simulink model "crne"  (R2018b)
settings: Solver=VariableStepAuto  StartTime=0.0  StopTime=7  RelTol=1e-3
undefined symbols (not defined in the file): eff_g_y, eff_m_y, J_phi, Kg_y, Kt_y, mp, r_y_reel
libraries: fuzblock x1
settings Model: Creator=EMiR  LastModifiedBy=EMiR

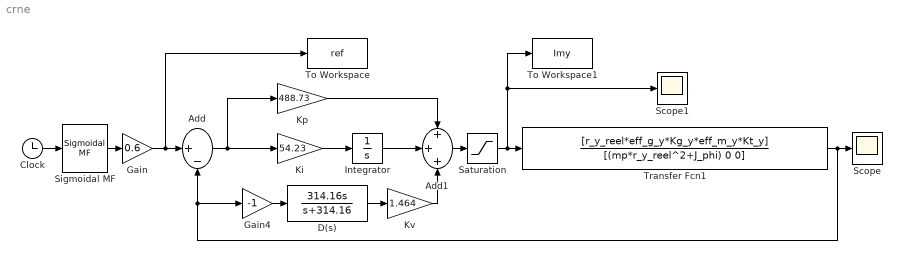
== system crne ==
  Add : Sum  Inputs=|+-
  Add1 : Sum  Inputs=+++
  Clock : Clock
      settings: Decimation=7
  D(s) : TransferFcn  Numerator=[314.16 0]  Denominator=[1 314.16]
  Gain : Gain  Gain=0.6
  Gain4 : Gain  Gain=-1
  Integrator : Integrator
  Ki : Gain  Gain=54.23
  Kp : Gain  Gain=488.73
  Kv : Gain  Gain=1.464
  Saturation : Saturate  UpperLimit=7  LowerLimit=-7
  Scope : Scope
  Scope1 : Scope
  Sigmoidal MF : fuzblock/Membership  Functions/Sigmoidal MF  a=5  c=3
      settings: SourceProductName=Fuzzy Logic Toolbox  SourceProductBaseCode=FL
  To Workspace : ToWorkspace  VariableName=ref  SampleTime=-1
  To Workspace1 : ToWorkspace  VariableName=Imy  SampleTime=-1
  Transfer Fcn1 : TransferFcn  Numerator=[r_y_reel*eff_g_y*Kg_y*eff_m_y*Kt_y]  Denominator=[(mp*r_y_reel^2+J_phi) 0 0]
  wires:
  Clock/1 -> Sigmoidal MF/1
  Sigmoidal MF/1 -> Gain/1
  Gain/1 -> Add/1, To Workspace/1
  Gain4/1 -> D(s)/1
  D(s)/1 -> Kv/1
  Ki/1 -> Integrator/1
  Integrator/1 -> Add1/2
  Kp/1 -> Add1/1
  Kv/1 -> Add1/3
  Add/1 -> Kp/1, Ki/1
  Transfer Fcn1/1 -> Scope/1, Add/2, Gain4/1
  Add1/1 -> Saturation/1
  Saturation/1 -> Scope1/1, To Workspace1/1, Transfer Fcn1/1
